simulink library "environmentSyntheticFlow_cl"  (R2020a)
settings: Solver=VariableStepAuto  StartTime=0.0  StopTime=10.0  RelTol=1e-3
undefined symbols (not defined in the file or in its folder): env, initializeBussesFromBlock
libraries: syntheticFlow_ul x4
settings Model: Creator=Ayaz  LastModifiedBy=Ayaz

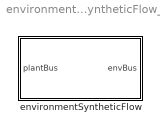
== system environmentSyntheticFlow_cl ==
  environmentSyntheticFlow : Subsystem  LoadFcn=initializeBussesFromBlock(gcb)  InitFcn=initializeBussesFromBlock(gcb)  StartFcn=initializeBussesFromBlock(gcb)  mask{en=env}
      mask prompts: en "Environment object"
      mask TypeOptions en: syntheticFlow/en | syntheticFlow1/en | syntheticFlow2/en | syntheticFlow3/en

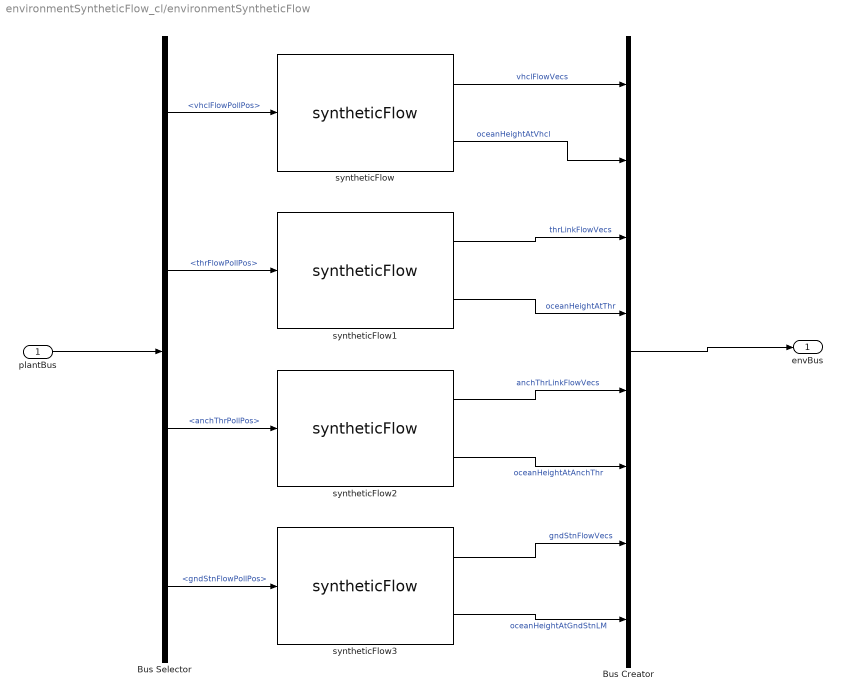
== system environmentSyntheticFlow_cl/environmentSyntheticFlow ==
  plantBus : Inport  OutDataTypeStr=Bus: plantBus
  Bus Creator : BusCreator  Inputs=8  OutDataTypeStr=Bus: envBus  NonVirtualBus=on
  Bus Selector : BusSelector  OutputSignals=vhclFlowPollPos,thrFlowPollPos,anchThrPollPos,gndStnFlowPollPos
  syntheticFlow{,1..3} (4 alike) : syntheticFlow_ul/syntheticFlow  en=en
  envBus : Outport  OutDataTypeStr=Bus: envBus  VectorParamsAs1DForOutWhenUnconnected=off
  wires:
  Bus Creator/1 -> envBus/1
  Bus Selector/2 -> syntheticFlow1/1  "<thrFlowPollPos>"
  syntheticFlow1/1 -> Bus Creator/3  "thrLinkFlowVecs"
  syntheticFlow1/2 -> Bus Creator/4  "oceanHeightAtThr"
  plantBus/1 -> Bus Selector/1
  syntheticFlow3/1 -> Bus Creator/7  "gndStnFlowVecs"
  syntheticFlow2/2 -> Bus Creator/6  "oceanHeightAtAnchThr"
  Bus Selector/3 -> syntheticFlow2/1  "<anchThrPollPos>"
  Bus Selector/4 -> syntheticFlow3/1  "<gndStnFlowPollPos>"
  syntheticFlow/2 -> Bus Creator/2  "oceanHeightAtVhcl"
  Bus Selector/1 -> syntheticFlow/1  "<vhclFlowPollPos>"
  syntheticFlow/1 -> Bus Creator/1  "vhclFlowVecs"
  syntheticFlow3/2 -> Bus Creator/8  "oceanHeightAtGndStnLM"
  syntheticFlow2/1 -> Bus Creator/5  "anchThrLinkFlowVecs"
